simulink model "Bouc_Wen_zdot"  (R2019a)
settings: Solver=VariableStepAuto  StartTime=0.0  StopTime=10.0  RelTol=1e-3
undefined symbols (not defined in the file): sigbuilder_block
settings Model: Creator=robertwright  LastModifiedBy=robertwright

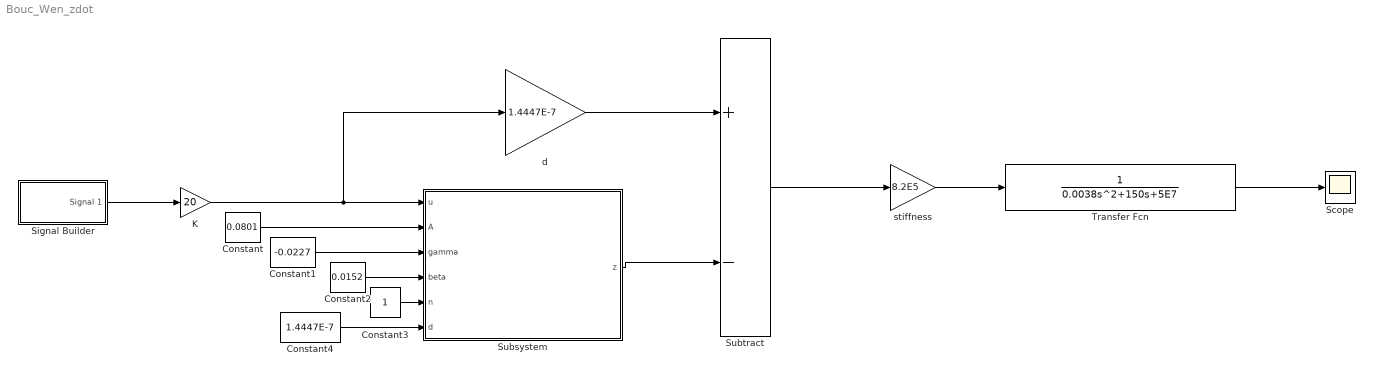
== system Bouc_Wen_zdot ==
  Constant : Constant  Value=0.0801
  Constant1 : Constant  Value=-0.0227
  Constant2 : Constant  Value=0.0152
  Constant3 : Constant
  Constant4 : Constant  Value=1.4447E-7
  K : Gain  Gain=20
  Scope : Scope
  Signal Builder : Subsystem  Tag=STV Subsys  LoadFcn=sigbuilder_block('load');  StartFcn=sigbuilder_block('start');  StopFcn=sigbuilder_block('stop');  ClipboardFcn=sigbuilder_block('clipboard');  mask(Sigbuilder block){tuvar=[0:10]}
      mask help: Simulink:masks:SigbuilderBlock_MD
      mask init:
      | if ~strcmp(get_param(bdroot(gcbh),'SimulationStatus'),'stopped') tuvar = sigbuilder_block('maskInit'); end
      settings: CopyFcn=sigbuilder_block('copy');  DeleteFcn=sigbuilder_block('delete');  ModelCloseFcn=sigbuilder_block('modelClose');  PreSaveFcn=sigbuilder_block('preSave');  PauseFcn=sigbuilder_block('pause');  ContinueFcn=sigbuilder_block('continue');  NameChangeFcn=sigbuilder_block('namechange');  OpenFcn=sigbuilder_block('open',[437.6 200 550.4 400 ]);  CloseFcn=sigbuilder_block('close');
      mask Display: plot(0, 0, 100, 100,[2, 2, 32, 32, 2], [68, 8, 8, 68, 68],[32, 2], [38, 38], [32, 19, 2],[53, 60, 44], [32, 17, 17, 2],[16, 16, 31, 31]);txt = getActiveGroup(gcbh);text(2, 100, txt,'verticalAlignment', 'top');
  Subsystem : Subsystem
  Subtract : Sum  Inputs=+-
  Transfer Fcn : TransferFcn  Denominator=[0.0038,150,5E7]
  d : Gain  Gain=1.4447E-7
  stiffness : Gain  Gain=8.2E5
  wires:
  Constant3/1 -> Subsystem/5(n)
  Constant2/1 -> Subsystem/4(beta)
  Constant1/1 -> Subsystem/3(gamma)
  Constant/1 -> Subsystem/2(A)
  Signal Builder/1(Signal 1) -> K/1
  K/1 -> d/1, Subsystem/1(u)
  Subsystem/1(z) -> Subtract/2
  d/1 -> Subtract/1
  Subtract/1 -> stiffness/1
  stiffness/1 -> Transfer Fcn/1
  Transfer Fcn/1 -> Scope/1
  Constant4/1 -> Subsystem/6(d)

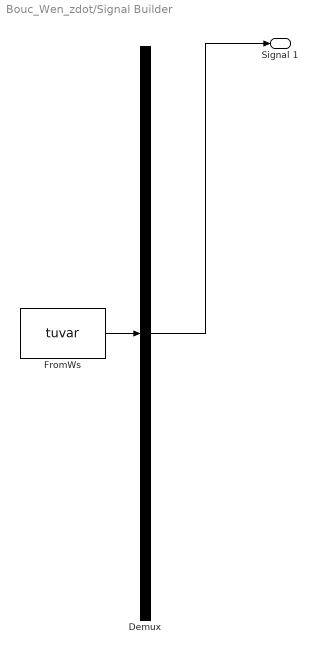
== system Bouc_Wen_zdot/Signal Builder ==
  Demux : Demux  Tag=STV Demux  Outputs=1
  FromWs : FromWorkspace  Tag=STV FromWs  VariableName=tuvar  SampleTime=0
      SigBuilderData=|
      | common.afterFinalStr = 'Extrapolate'
      | common.sampleTime = 0
      | dataSet.timeRange = [0 10]
      | dataSet.name = 'Group 1'
      | sbobj.Groups.Name = 'Group 1'
      | sbobj.Groups.Signals.Name = 'Signal 1'
      | sbobj.Groups.Signals.XData = [0 0.0331016219795 0.066203243959 0.0993048659384 0.132406487918 0.165508109897 0.198609731877 0.231711353856 0.264812975836 0.297914597815 0.331016219795 0.364117841774 ... (304 elements, 1x304)]
      | sbobj.Groups.Signals.YData = [0 0.324699469205 0.61421271269 0.837166478263 0.969400265939 0.996584493007 0.915773326655 0.735723910673 0.475947393037 0.164594590281 -0.164594590281 -0.475947393037 ... (304 elements, 1x304)]
  Signal 1 : Outport  Tag=STV Outport
  wires:
  Demux/1 -> Signal 1/1
  FromWs/1 -> Demux/1

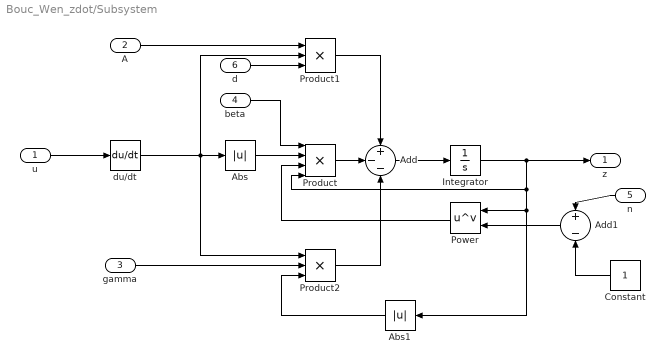
== system Bouc_Wen_zdot/Subsystem ==
  u : Inport
  A : Inport  Port=2
  gamma : Inport  Port=3
  beta : Inport  Port=4
  n : Inport  Port=5
  d : Inport  Port=6
  Abs : Abs
  Abs1 : Abs
  Add : Sum  Inputs=+--
  Add1 : Sum  Inputs=+-
  Constant : Constant
  Integrator : Integrator
  Power : Math  Operator=pow  SaturateOnIntegerOverflow=on
  Product : Product  Inputs=4
  Product1 : Product  Inputs=3
  Product2 : Product  Inputs=3
  du/dt : Derivative
  z : Outport
  wires:
  Product/1 -> Add/2
  beta/1 -> Product/1
  Product1/1 -> Add/1
  gamma/1 -> Product2/2
  Power/1 -> Product/3
  Abs1/1 -> Product2/3
  Constant/1 -> Add1/2
  Add/1 -> Integrator/1
  Product2/1 -> Add/3
  n/1 -> Add1/1
  Abs/1 -> Product/2
  A/1 -> Product1/1
  du/dt/1 -> Product2/1, Abs/1, Product1/2
  u/1 -> du/dt/1
  Integrator/1 -> z/1, Abs1/1, Power/1, Product/4
  Add1/1 -> Power/2
  d/1 -> Product1/3
